simulink model "simDc"  (R2024a)
settings: Solver=ode45  StartTime=0.0  StopTime=simTimeStop  FixedStep=0.001  RelTol=1e-3
undefined symbols (not defined in the file or in its folder): J, Kg, Mgr, Ra, simStepAmp
settings Model: Creator=simon  LastModifiedBy=simon
settings RTWCC: GPUComputeCapability=3.5

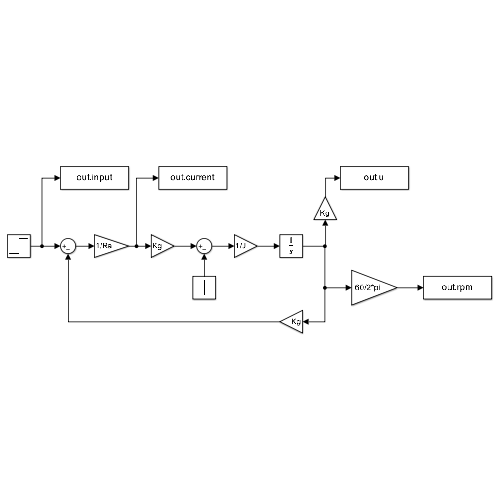
[thumbnail: Simulink's stored preview of the top-level diagram]
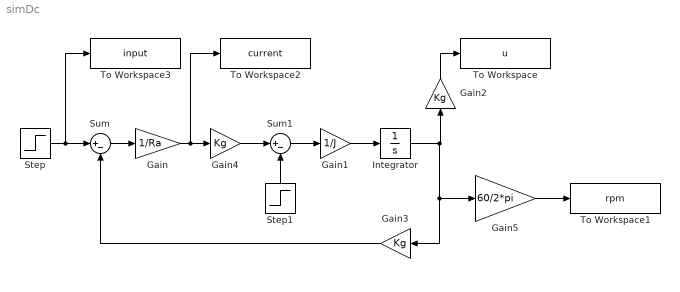
== system simDc ==
  Gain : Gain  Gain=1/Ra
  Gain1 : Gain  Gain=1/J
  Gain2 : Gain  Gain=Kg
  Gain3 : Gain  Gain=Kg
  Gain4 : Gain  Gain=Kg
  Gain5 : Gain  Gain=60/2*pi
  Integrator : Integrator
  Step : Step  Time=0  After=simStepAmp  SampleTime=0
  Step1 : Step  Time=0  After=Mgr  SampleTime=0
  Sum : Sum  Inputs=|+-
  Sum1 : Sum  Inputs=|+-
  To Workspace : ToWorkspace  VariableName=u  SaveFormat=Timeseries  SampleTime=-1
  To Workspace1 : ToWorkspace  VariableName=rpm  SaveFormat=Timeseries  SampleTime=-1
  To Workspace2 : ToWorkspace  VariableName=current  SaveFormat=Timeseries  SampleTime=-1
  To Workspace3 : ToWorkspace  VariableName=input  SaveFormat=Timeseries  SampleTime=-1
  wires:
  Step/1 -> To Workspace3/1, Sum/1
  Sum/1 -> Gain/1
  Gain/1 -> To Workspace2/1, Gain4/1
  Step1/1 -> Sum1/2
  Sum1/1 -> Gain1/1
  Gain1/1 -> Integrator/1
  Integrator/1 -> Gain3/1, Gain5/1, Gain2/1
  Gain3/1 -> Sum/2
  Gain4/1 -> Sum1/1
  Gain2/1 -> To Workspace/1
  Gain5/1 -> To Workspace1/1
